simulink model "XMC_FFT2D_HDL_AIE"  (R2024a)
settings: Solver=FixedStepDiscrete  StartTime=0.0  StopTime=256*256*2  RelTol=1e-3
PreLoadFcn:
  | MRIDemo_PreloadFcn;
  | 
  | % configure hardware specifics information
  | clock_frequency = 150e6;
  | 
  | % corner bender info
  | clk = clock_frequency; %Hz
  | Tclk = 1/clk;
  | L2M = 8; % L2M=log2(M)
  | L2N = 8; % L2N=log2(N)
  | M = 2^L2M;
  | N = 2^L2N;
  | SSR = 1;
InitFcn:
  | xlEvaluateHDLBlocks('XMC_FFT2D_HDL_AIE')
undefined symbols (not defined in the file): c, gray, None, S, vsva2197, xcvc1902
libraries: hdlBasic x137, aieUtilities x3, aieDSP x2, dspxfrm3 x2, dspsrcs4 x2, simulink x1, vmcUtilities x1
(part 1 of 2)
settings Model: PauseTimes=256*254  SnapshotBufferSize=1000  SnapshotInterval=1  Creator=mmi  LastModifiedBy=sdegala
settings SolverCC: AlgebraicLoopSolver=TrustRegion
settings DataIOCC: ReturnWorkspaceOutputs=off
settings DebuggingCC: UnconnectedInputMsg=warning  UnconnectedOutputMsg=warning  UnconnectedLineMsg=warning  ArithmeticOperatorsInVariantConditions=warning
settings ModelReferenceCC: EnableRefExpFcnMdlSchedulingChecks=on
settings SFSimCC: SimUseLocalCustomCode=off  CustomCodeUndefinedFunction=UseInterfaceOnly
settings RTWCC: RTWUseLocalCustomCode=off  GPUComputeCapability=3.5  DLArmComputeVersion=19.05

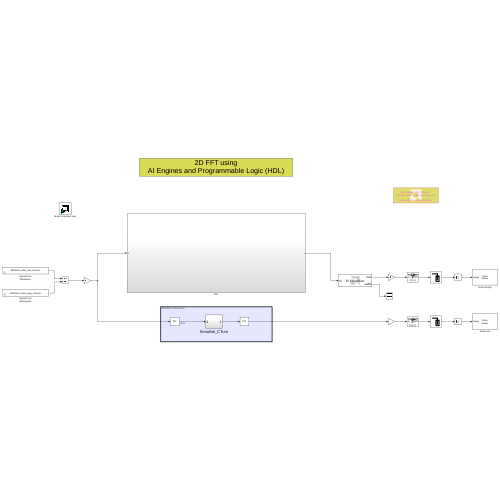
[thumbnail: Simulink's stored preview of the top-level diagram]
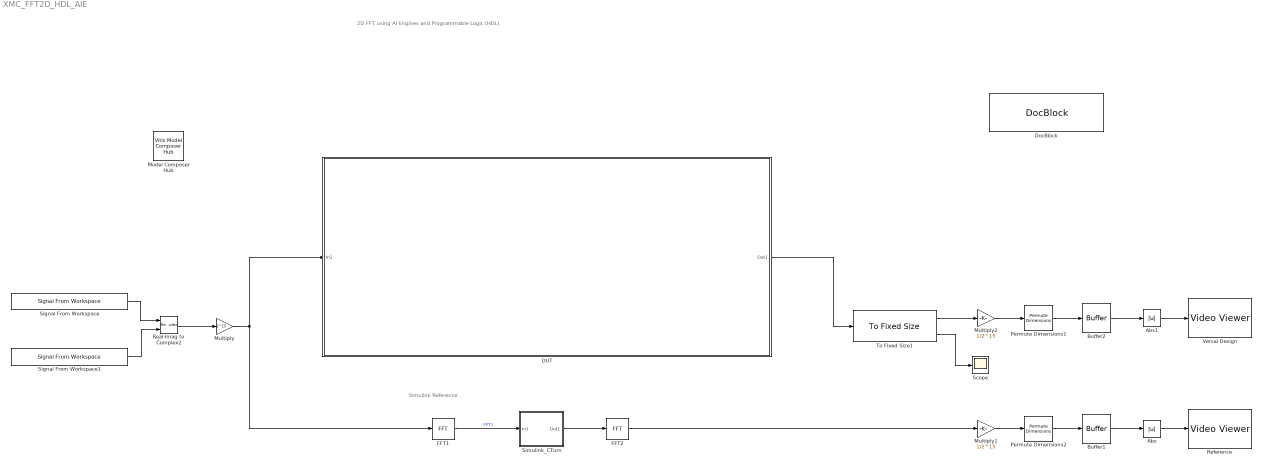
== system XMC_FFT2D_HDL_AIE ==
  note: Simulink Reference
  note: 2D FFT using
      | AI Engines and Programmable Logic (HDL)
  Abs : Abs  SaturateOnIntegerOverflow=off
  Abs1 : Abs  SaturateOnIntegerOverflow=off
  Buffer1 : Buffer  N=256  OutputFrames=off
  Buffer2 : Buffer  N=256  OutputFrames=off
  DUT : Subsystem
  DocBlock : simulink/Model-Wide Utilities/DocBlock  DocumentType=Text  mask(DocBlock){}
      content=|
      | ///////////////////////////////////////////////////////////////////////////
      | // Copyright 2021 Xilinx
      | //
      | // Licensed under the Apache License, Version 2.0 (the "License");
      | // you may not use this file except in compliance with the License.
      | // You may obtain a copy of the License at
      | //
      | // http://www.apache.org/licenses/LICENSE-2.0
      | //
      | // Unless required by applicable law or agreed to in writing, software
      | // distributed under the License is distributed on an "AS IS" BASIS,
      | // WITHOUT WARRANTIES OR CONDITIONS OF ANY KIND, either express or implied.
      | // See the License for the specific language governing permissions and
      | // limitations under the License.
      | ///////////////////////////////////////////////////////////////////////////
      mask Display:
      | xmcDrawBlockIcon();
      | disp(['{\fontsize{10pt}(c) Copyright 2021' ' Xilinx, Inc.}\newline \newline '],'texmode','on');
      | disp('{\fontsize{10pt}Licensed under the Apache License 2.0}','texmode','on');
      | disp('\newline \newline \newline{\fontsize{10pt}Double Click for Copyright Notice}','texmode','on');
  FFT1 : dspxfrm3/FFT  FFTImplementation=Auto  CompMethod=Table lookup  TableOpt=NEW  TableOptActive=Speed  BitRevOrder=off  Normalize=off  InheritFFTLength=on  FFTLength=64  WrapInput=on  roundingMode=Floor  overflowMode=off  firstCoeffDataTypeStr=Inherit: Same word length as input  firstCoeffLastDataTypeStr=Inherit: Same word length as input  prodOutputMode=Binary point scaling  prodOutputWordLength=32  prodOutputFracLength=0  prodOutputDataTypeStr=fixdt(1,32,0)  prodOutputLastDataTypeStr=fixdt(1,32,0)  accumMode=Binary point scaling  accumWordLength=48  accumFracLength=0  accumDataTypeStr=fixdt(1,48,0)  accumLastDataTypeStr=fixdt(1,48,0)  outputMode=Binary point scaling  outputWordLength=16  outputFracLength=0  outputDataTypeStr=fixdt(1,16,0)  outputMin=[]  outputMax=[]  outputLastDataTypeStr=fixdt(1,16,0)
  FFT2 : dspxfrm3/FFT  FFTImplementation=Auto  CompMethod=Table lookup  TableOpt=NEW  TableOptActive=Speed  BitRevOrder=off  Normalize=off  InheritFFTLength=on  FFTLength=64  WrapInput=on  roundingMode=Floor  overflowMode=off  firstCoeffDataTypeStr=Inherit: Same word length as input  firstCoeffLastDataTypeStr=Inherit: Same word length as input  prodOutputMode=Binary point scaling  prodOutputWordLength=32  prodOutputFracLength=0  prodOutputDataTypeStr=fixdt(1,32,0)  prodOutputLastDataTypeStr=fixdt(1,32,0)  accumMode=Binary point scaling  accumWordLength=48  accumFracLength=0  accumDataTypeStr=fixdt(1,48,0)  accumLastDataTypeStr=fixdt(1,48,0)  outputMode=Binary point scaling  outputWordLength=16  outputFracLength=0  outputDataTypeStr=fixdt(1,16,0)  outputMin=[]  outputMax=[]  outputLastDataTypeStr=fixdt(1,16,0)
  Model Composer Hub : vmcUtilities/Vitis Model Composer Hub  Tag=genX  CodeGeneration=off  SubsystemName=hdl_corner_turn  BlockHierPath=XMC_FFT2D_HDL_AIE/DUT  CompilationType=VitisCompilation  SubsystemType=DUTNode  ExportTypeV2=GenXO  AIEArrayConfig=Use entire AIE array  StartColumn=1  NumberOfColumns=1  TargetDirectory=./code  exportDesign=on  analyzeDesign=off  validateDesignOnHw=off  ExportType=Vitis Subsystem  IpVendor=xilinx.com  IpLibrary=hls  IpVersion=1.0  IpHWLanguage=Verilog  AieCompilerOptions={}  AieSimulatorOptions={}  CreateTestbench=off  TestbenchStackSize=10  RunRtlSim=off  RunCSim=off  RunAieSim=on  AieSimTimeout=50000  RunAieSimProfiling=off  LaunchVitisAnalyzer=off  PlotOutput=off  RunX86Sim=off  X86SimTimeout=10  GenHwImage=off  GenLibadfXo=on  GenHwValidationCode=on  PlatformType=Not Specified  HwSystemType=Baremetal  HwValidationTarget=hw  ProjDevice=xcvc1902-vsva2197-1LP-e-S  ProjDevicePart=xcvc1902-vsva2197-1LP-e-S  AIEType=AIE  SamplePeriod=-1  ClockFrequency=200  DataPathParallelism=1  xilinxfamily=versalaicore  part=xcvc1902  speed=-1LP-e-S  package=vsva2197  directory=./code/ip/hdl_corner_turn/src  testbench=on  incr_netlist=off  synthesis_tool=Vivado  clock_wrapper=Clock Enables  dbl_ovrd=According to Block Masks  dcm_input_clock_period=10  sysclk_period=10  simulink_period=1  eval_field=0  IPInfoJsonString="{\"DUTSubsystemName\":\"DUT\",\"HDLSubsystem\":{\"SubsystemName\":\"hdl_corner_turn\",\"IPName\":\"XMC_FFT2D_HDL_AIE\",\"IPLibrary\":\"SysGen\",\"IPVendor\":\"User Company\",\"IPVersion\":\"1.0\",\"TargetDirectory\":\"./code\",\"SubsystemDir\":\"./code/ip/hdl_corner_turn\",\"FreqHz\":\"100000000\"},\"SubsystemTag\":\"DUTNode\",\"AIESubsystem\":{\"SubsystemName\":\"aie_fft\",\"TargetDirectory\":\"./code\",\"AIEArrayConfig\":\"Use entire AIE array\",\"StartColumn\":\"1\",\"NumberOfColumns\":\"1\"}}"  LogFileName=/proj/xhdhdstaff5/sdegala/Head1/HEAD/ModelComposer_Sept16/Vitis_Model_Composer/Examples/AIENGINE_plus_PL/AIE_HDL/FFT2D/code/model_composer.log  NThreads=4  IPConfigFile=/tmp/vmctmp-7771901812203365421/XMC_FFT2D_HDL_AIE_ipconfig.json
  Multiply : Gain  Gain=2^15  OutDataTypeStr=int16
  Multiply1 : Gain  Gain=1/2^15  OutDataTypeStr=single
  Multiply2 : Gain  Gain=1/2^15  OutDataTypeStr=single
  Permute Dimensions1 : PermuteDimensions
  Permute Dimensions2 : PermuteDimensions
  Real-Imag to Complex2 : RealImagToComplex
  Reference : VideoViewer  Description=Simulink MRI Display  colormapValue=gray(256)  FigPos=[1133 905 574 478]
  Scope : Scope
  Signal From Workspace : dspsrcs4/Signal From Workspace  X=MRIDemo_data_real_channel  Ts=1  nsamps=256  OutputAfterFinalValue=Setting to zero  ignoreOrWarnInputAndFrameLengths=off  OutputFrames=off
  Signal From Workspace1 : dspsrcs4/Signal From Workspace  X=MRIDemo_data_imag_channel  Ts=1  nsamps=256  OutputAfterFinalValue=Setting to zero  ignoreOrWarnInputAndFrameLengths=off  OutputFrames=off
  Simulink_CTurn : Subsystem
  To Fixed Size1 : aieUtilities/To Fixed Size  Mode=Produce a valid output signal  OutputSize=256  CopyMethod=Buffer samples to form output  HasStatusOutput=off
  Versal Design : VideoViewer  Description=Simulink MRI Display  colormapValue=gray(256)  FigPos=[1062 805 703 270]
  wires:
  Real-Imag to Complex2/1 -> Multiply/1
  Signal From Workspace/1 -> Real-Imag to Complex2/1
  Signal From Workspace1/1 -> Real-Imag to Complex2/2
  Multiply1/1 -> Permute Dimensions2/1
  Abs/1 -> Reference/1
  Permute Dimensions2/1 -> Buffer1/1
  Buffer1/1 -> Abs/1
  Multiply/1 -> DUT/1(In1), FFT1/1
  FFT1/1 -> Simulink_CTurn/1(In1)  "FFT1"
  FFT2/1 -> Multiply1/1
  Simulink_CTurn/1(Out1) -> FFT2/1
  Abs1/1 -> Versal Design/1
  Buffer2/1 -> Abs1/1
  Permute Dimensions1/1 -> Buffer2/1
  Multiply2/1 -> Permute Dimensions1/1
  To Fixed Size1/1 -> Multiply2/1
  To Fixed Size1/2 -> Scope/1
  DUT/1(Out1) -> To Fixed Size1/1

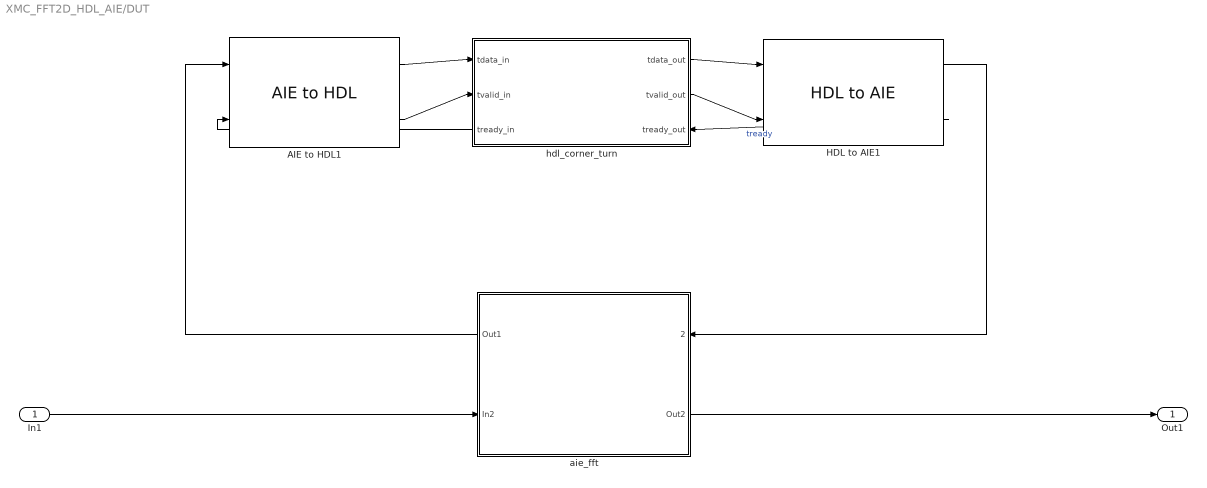
== system XMC_FFT2D_HDL_AIE/DUT ==
  In1 : Inport
  AIE to HDL1 : aieUtilities/AIE to HDL  OutDataType=uint32  OutSampleTime=1
      link override AIE to HDL_tready: inherit_from_input=on  hdl_port=on  rows=1  columns=1  UseAsDAC=off  DACChannel='1'  interface=None  automatic_assignment=on  address_offset=hex2dec('00')  intf_name=''  intf_description=''  timing_constraint=None  locs_specified=off  LOCs={}  io_standard={}
      link override AIE to HDL_tready: infoedit="Gateway out block.  Converts Xilinx fixed-point or floating-point type inputs into ouputs of type Simulink integer, single, double, or fixed-point.<br><br>Hardware notes:  In hardware these blocks become top level output ports or are discarded, depending on how they are configured."
  HDL to AIE1 : aieUtilities/HDL to AIE  InDataType=uint32  OutDataType=int16 (c)  OutSampleTime=1  SamplesPerFrame=256  RateReduceFactor=1  ManuallySpecifyOutSampleTime=on
  aie_fft : Subsystem
      settings: PortSchema="{\"entries\":[{\"content\":{\"sides\":[{\"content\":{\"connectorIds\":[\"Out2\",\"In1\"]},\"type\":\"ConnectorPlacement.EquallySpacedRectSide\",\"uuid\":\"ba116f73-e116-40b3-b2e5-304cba4df7e1\"},{\"content\":{\"connectorIds\":[\"In2\",\"Out1\"],\"side\":\"RIGHT\"},\"type\":\"ConnectorPlacement.EquallySpacedRectSide\",\"uuid\":\"f8ace37c-ffb0-4f56-a1b3-7eeef7565cfd\"},{\"content\":{\"connectorIds\":[],\"side\":\"TOP\"},\"type\":\"ConnectorPlacement.EquallySpacedRectSide\",\"uuid\":\"698d2e0a-1e8b-402b-bc99-cd34e1f9cd41\"}]},\"type\":\"ConnectorPlacement.EquallySpacedConnector\",\"uuid\":\"c9271cff-0d68-4ac4-bc57-5327e013a37e\"}],\"packageUris\":[\"http://schema.mathworks.com/mf0/Connector/R2020b\"],\"version\":\"1.0\"}"
  hdl_corner_turn : Subsystem
      settings: PortSchema="{\"entries\":[{\"content\":{\"sides\":[{\"content\":{\"connectorIds\":[\"In1\",\"In2\",\"Out3\"]},\"type\":\"ConnectorPlacement.EquallySpacedRectSide\",\"uuid\":\"096cfc4a-45cf-495e-9dad-5ec39c034de1\"},{\"content\":{\"connectorIds\":[\"Out1\",\"Out2\",\"In3\"],\"side\":\"RIGHT\"},\"type\":\"ConnectorPlacement.EquallySpacedRectSide\",\"uuid\":\"c2f58c53-17c1-4e0f-8fe6-4ca31b4ae7e7\"},{\"content\":{\"connectorIds\":[],\"side\":\"TOP\"},\"type\":\"ConnectorPlacement.EquallySpacedRectSide\",\"uuid\":\"fc0a0e48-62d9-4bc4-85b8-28883543f418\"}]},\"type\":\"ConnectorPlacement.EquallySpacedConnector\",\"uuid\":\"4d40c623-5fa9-4077-a912-8400e8a8f04d\"}],\"packageUris\":[\"http://schema.mathworks.com/mf0/Connector/R2020b\"],\"version\":\"1.0\"}"
  Out1 : Outport
  wires:
  hdl_corner_turn/3(tready_in) -> AIE to HDL1/2
  AIE to HDL1/2 -> hdl_corner_turn/2(tvalid_in)
  hdl_corner_turn/2(tvalid_out) -> HDL to AIE1/2
  aie_fft/1(Out2) -> Out1/1
  HDL to AIE1/2 -> hdl_corner_turn/3(tready_out)  "tready"
  In1/1 -> aie_fft/1(In2)
  AIE to HDL1/1 -> hdl_corner_turn/1(tdata_in)
  hdl_corner_turn/1(tdata_out) -> HDL to AIE1/1
  HDL to AIE1/1 -> aie_fft/2(" ")
  aie_fft/2(Out1) -> AIE to HDL1/1

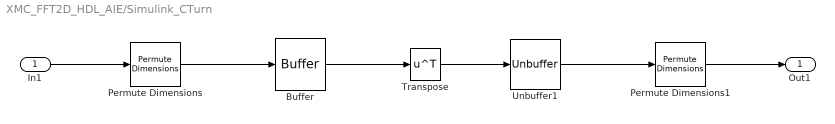
== system XMC_FFT2D_HDL_AIE/Simulink_CTurn ==
  In1 : Inport
  Buffer : Buffer  N=256  OutputFrames=off
  Permute Dimensions : PermuteDimensions
  Permute Dimensions1 : PermuteDimensions
  Transpose : Math  Operator=transpose  SignedPower=on
  Unbuffer1 : Unbuffer
  Out1 : Outport  VectorParamsAs1DForOutWhenUnconnected=off
  wires:
  Permute Dimensions/1 -> Buffer/1
  Transpose/1 -> Unbuffer1/1
  Buffer/1 -> Transpose/1
  In1/1 -> Permute Dimensions/1
  Unbuffer1/1 -> Permute Dimensions1/1
  Permute Dimensions1/1 -> Out1/1

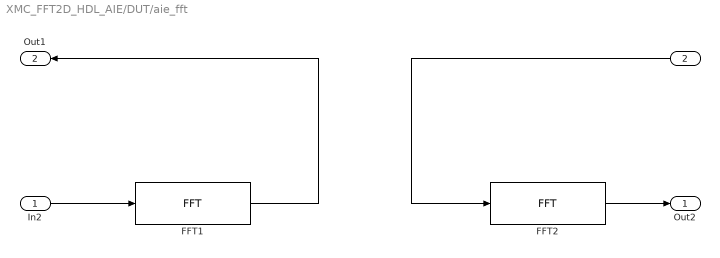
== system XMC_FFT2D_HDL_AIE/DUT/aie_fft ==
  In2 : Inport
  " " : Inport  Port=2
  FFT1 : aieDSP/FFT  AIE_VARIANT=1  data_type=cint16  data_out_type=cint16  twiddle_type=cint16  point_size=256  input_window_size=256  shift_val=0  rnd_mode=Round to positive infinity  sat_mode=0-None  ssr=1  twiddle_mode=0  use_ssr_widget_kernels=off  casc_length=1  transform_fft_nifft=1  TP_API=0  TP_DYN_PT_SIZE=0  blockJsonConstraints=[]  blockJsonConstraintsInternal="{\"type\":\"constraint\",\"constraintType\":\"coreUtilization\",\"sid\":\"82030:fft_graph.FFTwinproc.m_fftKernels[0]\",\"lhs\":{\"type\":\"runtimeRatio\",\"args\":{\"type\":\"kernel\",\"name\":\"XMC_FFT2D_HDL_AIE/Versal Desgin/aie_fft/FFT1\",\"sid\":\"82030:fft_graph.FFTwinproc.m_fftKernels[0]\"}},\"rhs\":{\"type\":\"evaluable\",\"expr\":\"0.9\",\"value\":0.9},\"equality\":true}"  spec=vmc_fft.json  SerializedMaskParamNames=[]  SerializedMaskParamValues=[]  SerializedMaskParamVisibilities=[]  block_type=FFT  SerializedMaskParamDataypes=uint|typename|typename|typename|uint|uint|uint|uint|uint|uint|uint|uint|uint|uint|uint|uint  SerializedMaskParamEnumStrArr=0|0|0|0|0|0|0|Round to positive infinity,Round to negative infinity,Round symmetrical to infinity,Round symmetrical to zero,Round convergent to even,Round convergent to odd|0-None,1-Asymmetric,3-Symmetric|0|0|0|0|0|0|0  SerializedMaskParamEnumValArr=0|0|0|0|0|0|0|2,3,4,5,6,7|0,1,3|0|0|0|0|0|0|0  SerializedMaskParamVectorArr=0|0|0|0|0|0|0|0|0|0|0|0|0|0|0|0  SerializedMaskParamKeys=AIE_VARIANT|TT_DATA|TT_OUT_DATA|TT_TWIDDLE|TP_POINT_SIZE|TP_WINDOW_VSIZE|TP_SHIFT|TP_RND|TP_SAT|TP_PARALLEL_POWER|TP_TWIDDLE_MODE|TP_USE_WIDGETS|TP_CASC_LEN|TP_FFT_NIFFT|TP_API|TP_DYN_PT_SIZE
  FFT2 : aieDSP/FFT  AIE_VARIANT=1  data_type=cint16  data_out_type=cint16  twiddle_type=cint16  point_size=256  input_window_size=256  shift_val=0  rnd_mode=Round to positive infinity  sat_mode=0-None  ssr=1  twiddle_mode=0  use_ssr_widget_kernels=off  casc_length=1  transform_fft_nifft=1  TP_API=0  TP_DYN_PT_SIZE=0  blockJsonConstraints=[]  blockJsonConstraintsInternal="{\"type\":\"constraint\",\"constraintType\":\"coreUtilization\",\"sid\":\"82031:fft_graph.FFTwinproc.m_fftKernels[0]\",\"lhs\":{\"type\":\"runtimeRatio\",\"args\":{\"type\":\"kernel\",\"name\":\"XMC_FFT2D_HDL_AIE/Versal Desgin/aie_fft/FFT2\",\"sid\":\"82031:fft_graph.FFTwinproc.m_fftKernels[0]\"}},\"rhs\":{\"type\":\"evaluable\",\"expr\":\"0.9\",\"value\":0.9},\"equality\":true}"  spec=vmc_fft.json  SerializedMaskParamNames=[]  SerializedMaskParamValues=[]  SerializedMaskParamVisibilities=[]  block_type=FFT  SerializedMaskParamDataypes=uint|typename|typename|typename|uint|uint|uint|uint|uint|uint|uint|uint|uint|uint|uint|uint  SerializedMaskParamEnumStrArr=0|0|0|0|0|0|0|Round to positive infinity,Round to negative infinity,Round symmetrical to infinity,Round symmetrical to zero,Round convergent to even,Round convergent to odd|0-None,1-Asymmetric,3-Symmetric|0|0|0|0|0|0|0  SerializedMaskParamEnumValArr=0|0|0|0|0|0|0|2,3,4,5,6,7|0,1,3|0|0|0|0|0|0|0  SerializedMaskParamVectorArr=0|0|0|0|0|0|0|0|0|0|0|0|0|0|0|0  SerializedMaskParamKeys=AIE_VARIANT|TT_DATA|TT_OUT_DATA|TT_TWIDDLE|TP_POINT_SIZE|TP_WINDOW_VSIZE|TP_SHIFT|TP_RND|TP_SAT|TP_PARALLEL_POWER|TP_TWIDDLE_MODE|TP_USE_WIDGETS|TP_CASC_LEN|TP_FFT_NIFFT|TP_API|TP_DYN_PT_SIZE
  Out2 : Outport
  Out1 : Outport  Port=2
  wires:
  FFT2/1 -> Out2/1
  " "/1 -> FFT2/1
  FFT1/1 -> Out1/1
  In2/1 -> FFT1/1

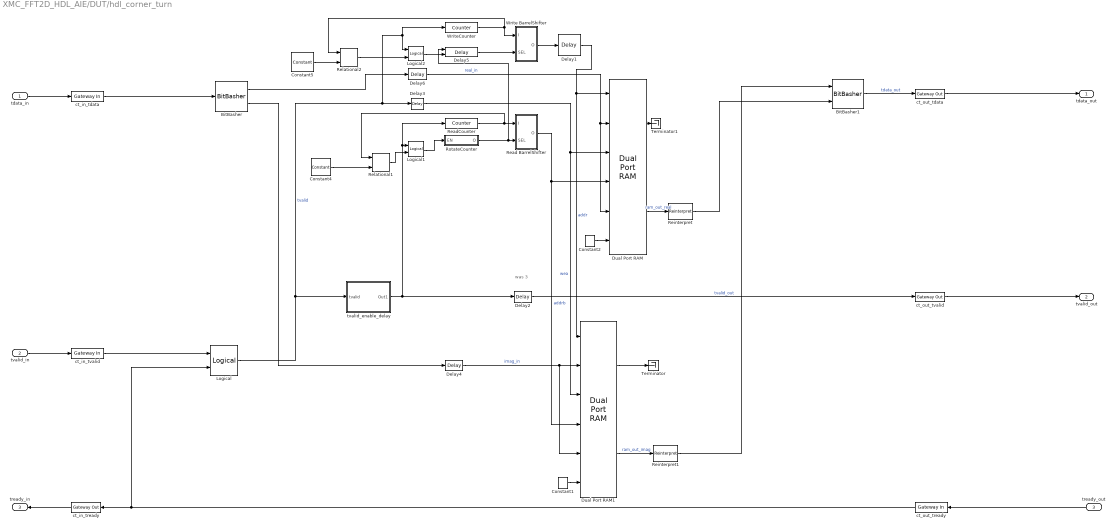
== system XMC_FFT2D_HDL_AIE/DUT/hdl_corner_turn ==
  note: was 3
  tdata_in : Inport
  tvalid_in : Inport  Port=2
  tready_out : Inport  Port=3
  BitBasher : hdlBasic/BitBasher  bitexpr=|  display_expr=off  sr_1=re  arith_type1="Signed  (2's comp)"  bin_pt1=0  sr_2=im  arith_type2="Signed  (2's comp)"  bin_pt2=0  sr_3=3  arith_type3=Unsigned  bin_pt3=0  sr_4=4  arith_type4=Unsigned  bin_pt4=0  XmcBlockStatus=1  maskContainerNames=group1  block_type=bitbasher  block_config=sysgen:BitBasher_config
      | re={cplx_in[15:0]};
      | im={cplx_in[31:16]};
  BitBasher1 : hdlBasic/BitBasher  bitexpr=cplx_out={im[15:0], re[15:0]};  display_expr=off  sr_1=cplx_out  arith_type1=Unsigned  bin_pt1=0  sr_2=im  arith_type2=Unsigned  bin_pt2=0  sr_3=3  arith_type3=Unsigned  bin_pt3=0  sr_4=4  arith_type4=Unsigned  bin_pt4=0  XmcBlockStatus=1  maskContainerNames=group1  block_type=bitbasher  block_config=sysgen:BitBasher_config
  Constant1 : hdlBasic/Constant  const=0  gui_display_data_type=Boolean  arith_type=Boolean  n_bits=40  bin_pt=20  preci_type=Single  exp_width=8  frac_width=24  explicit_period=off  period=1  XmcBlockStatus=1  maskContainerNames=tabcontainer1  block_type=constant  block_config=sysgen:Constant_config
  Constant2 : hdlBasic/Constant  const=0  gui_display_data_type=Boolean  arith_type=Boolean  n_bits=40  bin_pt=20  preci_type=Single  exp_width=8  frac_width=24  explicit_period=off  period=1  XmcBlockStatus=1  maskContainerNames=tabcontainer1  block_type=constant  block_config=sysgen:Constant_config
  Constant4 : hdlBasic/Constant  const=2^(L2M+L2N)-1  gui_display_data_type=Fixed-point  arith_type=Unsigned  n_bits=L2M+L2N  bin_pt=0  preci_type=Single  exp_width=8  frac_width=24  explicit_period=off  period=1  XmcBlockStatus=1  maskContainerNames=tabcontainer1  block_type=constant  block_config=sysgen:Constant_config
  Constant5 : hdlBasic/Constant  const=2^(L2M+L2N)-1  gui_display_data_type=Fixed-point  arith_type=Unsigned  n_bits=L2M+L2N  bin_pt=0  preci_type=Single  exp_width=8  frac_width=24  explicit_period=off  period=1  XmcBlockStatus=1  maskContainerNames=tabcontainer1  block_type=constant  block_config=sysgen:Constant_config
  Delay1 : hdlBasic/Delay  rst=off  en=off  latency=1  reg_retiming=off  XmcBlockStatus=1  maskContainerNames=group1  block_type=delay  block_config=sysgen:Delay_config
  Delay2 : hdlBasic/Delay  rst=off  en=off  latency=3  reg_retiming=off  XmcBlockStatus=1  maskContainerNames=group1  block_type=delay  block_config=sysgen:Delay_config
  Delay3 : hdlBasic/Delay  rst=off  en=off  latency=2  reg_retiming=off  XmcBlockStatus=1  maskContainerNames=group1  block_type=delay  block_config=sysgen:Delay_config
  Delay4 : hdlBasic/Delay  rst=off  en=off  latency=2  reg_retiming=off  XmcBlockStatus=1  maskContainerNames=group1  block_type=delay  block_config=sysgen:Delay_config
  Delay5 : hdlBasic/Delay  rst=off  en=on  latency=1  reg_retiming=off  XmcBlockStatus=1  maskContainerNames=group1  block_type=delay  block_config=sysgen:Delay_config
  Delay6 : hdlBasic/Delay  rst=off  en=off  latency=2  reg_retiming=off  XmcBlockStatus=1  maskContainerNames=group1  block_type=delay  block_config=sysgen:Delay_config
  Dual Port RAM : hdlBasic/Dual Port RAM  depth=2^L2M*2^L2N  initVector=zeros(2^L2M*2^L2N,1)  distributed_mem=Block RAM  init_a=0  init_b=0  rst_a=off  rst_b=off  en_a=off  en_b=off  latency=2  write_mode_A=Read After Write  write_mode_B=Read After Write  explicit_period=[]  period=[]  simulation_type=fast_sim  XmcBlockStatus=1  maskContainerNames=tabcontainer1  block_type=dpram  block_config=sysgen:Dpram_config  optimize=Area
      settings: infoedit=[]
  Dual Port RAM1 : hdlBasic/Dual Port RAM  depth=2^L2M*2^L2N  initVector=zeros(2^L2M*2^L2N,1)  distributed_mem=Block RAM  init_a=0  init_b=0  rst_a=off  rst_b=off  en_a=off  en_b=off  latency=2  write_mode_A=Read After Write  write_mode_B=Read After Write  explicit_period=[]  period=[]  simulation_type=fast_sim  XmcBlockStatus=1  maskContainerNames=tabcontainer1  block_type=dpram  block_config=sysgen:Dpram_config  optimize=Area
      settings: infoedit=[]
  Logical : hdlBasic/Logical  logical_function=AND  inputs=2  en=off  latency=0  precision=Full  arith_type=Unsigned  n_bits=16  bin_pt=0  align_bp=on  overflow=[]  quantization=[]  XmcBlockStatus=1  maskContainerNames=tabcontainer1  block_type=logical  block_config=sysgen:Logical_config
  Logical1 : hdlBasic/Logical  logical_function=AND  inputs=2  en=off  latency=0  precision=Full  arith_type=Unsigned  n_bits=16  bin_pt=0  align_bp=on  overflow=[]  quantization=[]  XmcBlockStatus=1  maskContainerNames=tabcontainer1  block_type=logical  block_config=sysgen:Logical_config
  Logical2 : hdlBasic/Logical  logical_function=AND  inputs=2  en=off  latency=0  precision=Full  arith_type=Unsigned  n_bits=16  bin_pt=0  align_bp=on  overflow=[]  quantization=[]  XmcBlockStatus=1  maskContainerNames=tabcontainer1  block_type=logical  block_config=sysgen:Logical_config
  Read BarrelShifter : Subsystem  mask{barrel_length=L2M+L2N}
      mask prompts: barrel_length "Barrel Length"
      mask init:
      | %%%%%%%%%%%%%%%%%%%%%%%%%%%%%%%%%%%%%%%%%%%%%%%%%%%%%
      | % Parametric Barrel Shifter Mask Initialization Script
      | % 18DEC2017: Creation
      | %%%%%%%%%%%%%%%%%%%%%%%%%%%%%%%%%%%%%%%%%%%%%%%%%%%%%
      | this=gcb;
      | 
      | %%%%%%%%%%%%%%%%%%%%%%%%%%%%%%%%%%%%%%%%%%%%%%%%%%%%%
      | % Delete wires and certain blocks; retain IO ports so parent
      | % mask block will not require re-connection
      | %%%%%%%%%%%%%%%%%%%%%%%%%%%%%%%%%%%%%%%%%%%%%%%%%%%%%
      | 
      | % delete all blocks except for d1 and q1
      | allblocks = find_system(this, 'LookUnderMasks','on','SearchDepth',1);
      | 
      | ToKeep = {'I';'O';'SEL';'Mux';'RotateLeft1'};
      | 
      | %// add systemname to strings
      | ToKeep = strcat(repmat({[this  '/']},numel(ToKeep),1), ToKeep);
      | 
      | %// create mask
      | ToDelete = setdiff(allblocks,ToKeep);
      | %// filter out main system
      | ToDelete = setxor(ToDelete,this);
      | 
      | cellfun(@(x) delete_block(x),ToDelete)
      | 
      | % delete lines
      | L = find_system(this,'LookUnderMasks','on','SearchDepth',1,'FindAll','on','type','line');
      | delete_line(L(1:end));
      | 
      | %%%%%%%%%%%%%%%%%%%%%%%%%%%%%%%%%%%%%%%%%%%%%%%%%%%%%%
      | % instantiate RotateLeft blocks and configure
      | %%%%%%%%%%%%%%%%%%%%%%%%%%%%%%%%%%%%%%%%%%%%%%%%%%%%%%
      | blockName1 = strcat(this,'/RotateLeft1');
      | x_loc = 70;
      | y_loc = 70;
      | for i = 2:barrel_length-1
      |     blockName = strcat(this,'/RotateLeft',num2str(i));
      |     blockHandle = add_block(blockName1,blockName, 'position',[x_loc,y_loc,x_loc+60,y_loc+20], ...
      |         'NB',num2str(i));
      |     y_loc = y_loc + 40;
      | end
      | 
      | %%%%%%%%%%%%%%%%%%%%%%%%%%%%%%%%%%%%%%%%%%%%%%%%%%%%%%
      | % Set mux parameters
      | %%%%%%%%%%%%%%%%%%%%%%%%%%%%%%%%%%%%%%%%%%%%%%%%%%%%%%
      | 
      | myMux = strcat(this,'/Mux');
      | set_param(myMux, 'inputs', barrel_length-2);
      | 
      | %%%%%%%%%%%%%%%%%%%%%%%%%%%%%%%%%%%%%%%%%%%%%%%%%%%%%%
      | % wires
      | %%%%%%%%%%%%%%%%%%%%%%%%%%%%%%%%%%%%%%%%%%%%%%%%%%%%%%
      | 
      | % RotateLeft to mux
      | 
      | h_myMux = get_param(myMux,'PortHandles');
      | 
      | for i = 1:barrel_length-1  
      |   blockName = strcat(this,'/RotateLeft',num2str(i));
      |   h_RotateLeft =  get_param(blockName,'PortHandles');
      |   add_line(this,{h_RotateLeft.Outport} ,{h_myMux.Inport(i+2)},'autorouting','on');
      | end
      | 
      | % mux to outport
      | h_myOutport = get_param(strcat(this,'/O'), 'PortHandles');
      | 
      | add_line(this,{h_myMux.Outport} ,{h_myOutport.Inport},'autorouting','on');
      | 
      | % inport to RotateLeft
      | h_myInport = get_param(strcat(this,'/I'), 'PortHandles');
      | 
      | for i = 1:barrel_length-1  
      |   blockName = strcat(this,'/RotateLeft',num2str(i));
      |   h_RotateLeft =  get_param(blockName,'PortHandles');
      |   add_line(this,{h_myInport.Outport} ,{h_RotateLeft.Inport},'autorouting','on');
      | end
      | 
      | % inport to mux
      | add_line(this,{h_myInport.Outport} ,{h_myMux.Inport(2)},'autorouting','on');
      | 
      | % SEL to mux
      | h_mySEL = get_param(strcat(this,'/SEL'), 'PortHandles');
      | add_line(this,{h_mySEL.Outport} ,{h_myMux.Inport(1)},'autorouting','on');
  ReadCounter : hdlBasic/Counter  cnt_type=Free running  cnt_to=Inf  operation=Up  start_count=0  cnt_by_val=1  arith_type=Unsigned  n_bits=L2M+L2N  bin_pt=0  load_pin=off  rst=off  en=on  explicit_period=Explicit  period=1  use_behavioral_HDL=off  implementation=Fabric  XmcBlockStatus=1  maskContainerNames=group1  block_type=counter  block_config=sysgen:Counter_config  block_width=531  block_height=1023
  Reinterpret : hdlBasic/Reinterpret  force_arith_type=on  arith_type=Unsigned  force_bin_pt=off  bin_pt=0  XmcBlockStatus=1  maskContainerNames=group1  block_type=reinterpret  block_config=sysgen:Reinterpret_config
  Reinterpret1 : hdlBasic/Reinterpret  force_arith_type=on  arith_type=Unsigned  force_bin_pt=off  bin_pt=0  XmcBlockStatus=1  maskContainerNames=group1  block_type=reinterpret  block_config=sysgen:Reinterpret_config
  Relational1 : hdlBasic/Relational  mode=a=b  op_type=Bool  en=off  latency=0  XmcBlockStatus=1  maskContainerNames=tabcontainer1  block_type=relational  block_config=sysgen:Relational_config
  Relational2 : hdlBasic/Relational  mode=a=b  op_type=Bool  en=off  latency=0  XmcBlockStatus=1  maskContainerNames=tabcontainer1  block_type=relational  block_config=sysgen:Relational_config
  RotateCounter : Subsystem  mask{L2M=L2M, L2N=L2N}
  Terminator : Terminator
  Terminator1 : Terminator
  Write BarrelShifter : Subsystem  mask{barrel_length=L2M+L2N}
      mask prompts: barrel_length "Barrel Length"
      mask init: same as XMC_FFT2D_HDL_AIE/DUT/hdl_corner_turn/Read BarrelShifter
  WriteCounter : hdlBasic/Counter  cnt_type=Free running  cnt_to=Inf  operation=Up  start_count=0  cnt_by_val=1  arith_type=Unsigned  n_bits=L2M+L2N  bin_pt=0  load_pin=off  rst=off  en=on  explicit_period=Explicit  period=1  use_behavioral_HDL=off  implementation=Fabric  XmcBlockStatus=1  maskContainerNames=group1  block_type=counter  block_config=sysgen:Counter_config  block_width=531  block_height=1023
  ct_in_tdata : hdlBasic/Gateway In  gui_display_data_type=Fixed-point  arith_type=Unsigned  n_bits=32  bin_pt=0  preci_type=Single  exp_width=8  frac_width=24  rows=1  columns=1  quantization="Round  (unbiased: +/- Inf)"  overflow=Saturate  period=1  UseAsADC=off  ADCChannel='1'  interface=None  automatic_assignment=on  address_offset=hex2dec('00')  intf_name=''  intf_description=''  default_value=0  timing_constraint=None  locs_specified=off  LOCs={}  io_standard={}  inherit_from_input=off  hdl_port=on  XmcBlockStatus=1  maskContainerNames=group4  block_type=gatewayin  block_config=sysgen:gateway_in_config  block_width_w=590  block_height_w=620  block_width=640  block_height=850
  ct_in_tready : hdlBasic/Gateway Out  inherit_from_input=on  bool_to_boolean=off  hdl_port=on  rows=1  columns=1  UseAsDAC=off  DACChannel='1'  interface=None  automatic_assignment=on  address_offset=hex2dec('00')  intf_name=''  intf_description=''  timing_constraint=None  locs_specified=off  LOCs={}  io_standard={}  XmcBlockStatus=1  maskContainerNames=group4  block_type=gatewayout  block_config=sysgen:gateway_out_config  block_width_w=590  block_height_w=620  block_width=620  block_height=750
  ct_in_tvalid : hdlBasic/Gateway In  gui_display_data_type=Boolean  arith_type=Boolean  n_bits=16  bin_pt=14  preci_type=Single  exp_width=8  frac_width=24  rows=1  columns=1  quantization="Round  (unbiased: +/- Inf)"  overflow=Saturate  period=1  UseAsADC=off  ADCChannel='1'  interface=None  automatic_assignment=on  address_offset=hex2dec('00')  intf_name=''  intf_description=''  default_value=0  timing_constraint=None  locs_specified=off  LOCs={}  io_standard={}  inherit_from_input=off  hdl_port=on  XmcBlockStatus=1  maskContainerNames=group4  block_type=gatewayin  block_config=sysgen:gateway_in_config  block_width_w=590  block_height_w=620  block_width=640  block_height=850
  ct_out_tdata : hdlBasic/Gateway Out  inherit_from_input=on  bool_to_boolean=off  hdl_port=on  rows=1  columns=1  UseAsDAC=off  DACChannel='1'  interface=None  automatic_assignment=on  address_offset=hex2dec('00')  intf_name=''  intf_description=''  timing_constraint=None  locs_specified=off  LOCs={}  io_standard={}  XmcBlockStatus=1  maskContainerNames=group4  block_type=gatewayout  block_config=sysgen:gateway_out_config  block_width_w=590  block_height_w=620  block_width=620  block_height=750
  ct_out_tready : hdlBasic/Gateway In  gui_display_data_type=Boolean  arith_type=Boolean  n_bits=16  bin_pt=14  preci_type=Single  exp_width=8  frac_width=24  rows=1  columns=1  quantization="Round  (unbiased: +/- Inf)"  overflow=Saturate  period=1  UseAsADC=off  ADCChannel='1'  interface=None  automatic_assignment=on  address_offset=hex2dec('00')  intf_name=''  intf_description=''  default_value=0  timing_constraint=None  locs_specified=off  LOCs={}  io_standard={}  inherit_from_input=off  hdl_port=on  XmcBlockStatus=1  maskContainerNames=group4  block_type=gatewayin  block_config=sysgen:gateway_in_config  block_width_w=590  block_height_w=620  block_width=640  block_height=850
  ct_out_tvalid : hdlBasic/Gateway Out  inherit_from_input=on  bool_to_boolean=off  hdl_port=on  rows=1  columns=1  UseAsDAC=off  DACChannel='1'  interface=None  automatic_assignment=on  address_offset=hex2dec('00')  intf_name=''  intf_description=''  timing_constraint=None  locs_specified=off  LOCs={}  io_standard={}  XmcBlockStatus=1  maskContainerNames=group4  block_type=gatewayout  block_config=sysgen:gateway_out_config  block_width_w=590  block_height_w=620  block_width=620  block_height=750
  tvalid_enable_delay : Subsystem
  tdata_out : Outport
  tvalid_out : Outport  Port=2
  tready_in : Outport  Port=3
  wires:
  Constant4/1 -> Relational1/2
  RotateCounter/1(O) -> Delay5/1, Read BarrelShifter/2(SEL)
  Constant1/1 -> Dual Port RAM1/6
  Reinterpret/1 -> BitBasher1/2
  Delay5/1 -> Write BarrelShifter/2(SEL)
  Relational1/1 -> Logical1/2
  Logical2/1 -> Delay5/2
  Constant5/1 -> Relational2/2
  ReadCounter/1 -> Read BarrelShifter/1(I), Relational1/1
  Dual Port RAM/2 -> Reinterpret/1  "ram_out_real"
  Read BarrelShifter/1(O) -> Dual Port RAM/4, Dual Port RAM1/4  "addrb"
  WriteCounter/1 -> Write BarrelShifter/1(I), Relational2/1
  Logical1/1 -> RotateCounter/1(EN)
  Delay4/1 -> Dual Port RAM1/5, Dual Port RAM1/2  "imag_in"
  BitBasher/2 -> Delay4/1
  Delay6/1 -> Dual Port RAM/5, Dual Port RAM/2  "real_in"
  tdata_in/1 -> ct_in_tdata/1
  Delay3/1 -> Dual Port RAM1/3, Dual Port RAM/3  "wea"
  Delay2/1 -> ct_out_tvalid/1  "tvalid_out"
  Dual Port RAM/1 -> Terminator1/1
  BitBasher1/1 -> ct_out_tdata/1  "tdata_out"
  Logical/1 -> Logical2/1, WriteCounter/1, Delay3/1, tvalid_enable_delay/1(tvalid)  "tvalid"
  Constant2/1 -> Dual Port RAM/6
  Dual Port RAM1/1 -> Terminator/1
  Write BarrelShifter/1(O) -> Delay1/1
  tvalid_in/1 -> ct_in_tvalid/1
  Relational2/1 -> Logical2/2
  Reinterpret1/1 -> BitBasher1/1
  tvalid_enable_delay/1(Out1) -> Delay2/1, ReadCounter/1, Logical1/1
  BitBasher/1 -> Delay6/1
  Delay1/1 -> Dual Port RAM/1, Dual Port RAM1/1  "addr"
  Dual Port RAM1/2 -> Reinterpret1/1  "ram_out_imag"
  tready_out/1 -> ct_out_tready/1
  ct_in_tdata/1 -> BitBasher/1
  ct_in_tvalid/1 -> Logical/1
  ct_out_tready/1 -> Logical/2, ct_in_tready/1
  ct_in_tready/1 -> tready_in/1
  ct_out_tvalid/1 -> tvalid_out/1
  ct_out_tdata/1 -> tdata_out/1

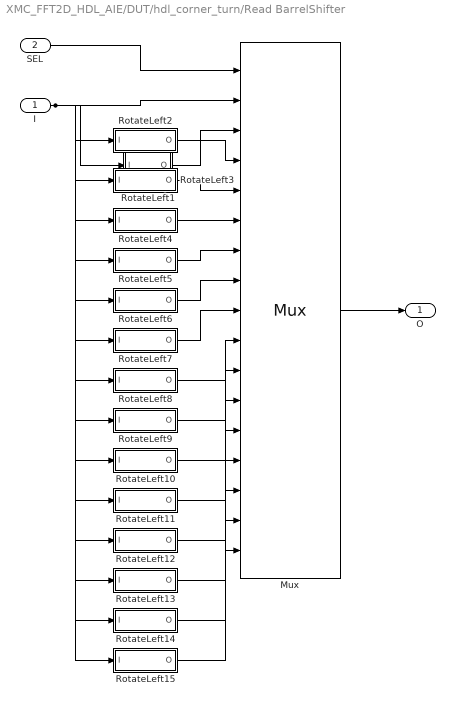
== system XMC_FFT2D_HDL_AIE/DUT/hdl_corner_turn/Read BarrelShifter ==
  I : Inport
  SEL : Inport  Port=2
  Mux : hdlBasic/Mux  inputs=16  en=off  latency=1  precision=Full  arith_type=Unsigned  n_bits=16  bin_pt=14  quantization=Truncate  overflow=Wrap  XmcBlockStatus=1  maskContainerNames=tabcontainer1  block_type=mux  block_config=sysgen:Mux_config
  RotateLeft1 : Subsystem  mask{NB=1, W=barrel_length}
      mask prompts: NB "Number of bits (cannot be 0):"; W "Width"
  RotateLeft10 : Subsystem  mask{NB=10, W=barrel_length}
      mask prompts: NB "Number of bits (cannot be 0):"; W "Width"
  RotateLeft11 : Subsystem  mask{NB=11, W=barrel_length}
      mask prompts: NB "Number of bits (cannot be 0):"; W "Width"
  RotateLeft12 : Subsystem  mask{NB=12, W=barrel_length}
      mask prompts: NB "Number of bits (cannot be 0):"; W "Width"
  RotateLeft13 : Subsystem  mask{NB=13, W=barrel_length}
      mask prompts: NB "Number of bits (cannot be 0):"; W "Width"
  RotateLeft14 : Subsystem  mask{NB=14, W=barrel_length}
      mask prompts: NB "Number of bits (cannot be 0):"; W "Width"
  RotateLeft15 : Subsystem  mask{NB=15, W=barrel_length}
      mask prompts: NB "Number of bits (cannot be 0):"; W "Width"
  RotateLeft2 : Subsystem  mask{NB=2, W=barrel_length}
      mask prompts: NB "Number of bits (cannot be 0):"; W "Width"
  RotateLeft3 : Subsystem  mask{NB=3, W=barrel_length}
      mask prompts: NB "Number of bits (cannot be 0):"; W "Width"
  RotateLeft4 : Subsystem  mask{NB=4, W=barrel_length}
      mask prompts: NB "Number of bits (cannot be 0):"; W "Width"
  RotateLeft5 : Subsystem  mask{NB=5, W=barrel_length}
      mask prompts: NB "Number of bits (cannot be 0):"; W "Width"
  RotateLeft6 : Subsystem  mask{NB=6, W=barrel_length}
      mask prompts: NB "Number of bits (cannot be 0):"; W "Width"
  RotateLeft7 : Subsystem  mask{NB=7, W=barrel_length}
      mask prompts: NB "Number of bits (cannot be 0):"; W "Width"
  RotateLeft8 : Subsystem  mask{NB=8, W=barrel_length}
      mask prompts: NB "Number of bits (cannot be 0):"; W "Width"
  RotateLeft9 : Subsystem  mask{NB=9, W=barrel_length}
      mask prompts: NB "Number of bits (cannot be 0):"; W "Width"
  O : Outport
  wires:
  RotateLeft1/1(O) -> Mux/3
  RotateLeft2/1(O) -> Mux/4
  RotateLeft3/1(O) -> Mux/5
  RotateLeft4/1(O) -> Mux/6
  RotateLeft5/1(O) -> Mux/7
  RotateLeft6/1(O) -> Mux/8
  RotateLeft7/1(O) -> Mux/9
  RotateLeft8/1(O) -> Mux/10
  RotateLeft9/1(O) -> Mux/11
  RotateLeft10/1(O) -> Mux/12
  RotateLeft11/1(O) -> Mux/13
  RotateLeft12/1(O) -> Mux/14
  RotateLeft13/1(O) -> Mux/15
  RotateLeft14/1(O) -> Mux/16
  RotateLeft15/1(O) -> Mux/17
  Mux/1 -> O/1
  I/1 -> RotateLeft1/1(I), RotateLeft2/1(I), RotateLeft3/1(I), RotateLeft4/1(I), RotateLeft5/1(I), RotateLeft6/1(I), RotateLeft7/1(I), RotateLeft8/1(I), RotateLeft9/1(I), RotateLeft10/1(I), RotateLeft11/1(I), RotateLeft12/1(I), RotateLeft13/1(I), RotateLeft14/1(I), RotateLeft15/1(I), Mux/2
  SEL/1 -> Mux/1

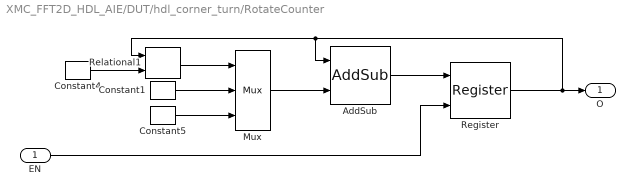
== system XMC_FFT2D_HDL_AIE/DUT/hdl_corner_turn/RotateCounter ==
  EN : Inport
  AddSub : hdlBasic/AddSub  mode=Addition  use_carryin=off  use_carryout=off  en=off  latency=0  precision=User Defined  arith_type=Unsigned  n_bits=ceil(log2(L2M+L2N))  bin_pt=0  quantization=Truncate  overflow=Wrap  use_behavioral_HDL=off  hw_selection=Fabric  pipelined=off  XmcBlockStatus=1  maskContainerNames=tabcontainer1  block_type=addsub  block_config=sysgen:Addsub_config
  Constant1 : hdlBasic/Constant  const=L2N  gui_display_data_type=Fixed-point  arith_type=Unsigned  n_bits=ceil(log2(L2M+L2N))  bin_pt=0  preci_type=Single  exp_width=8  frac_width=24  explicit_period=on  period=1  XmcBlockStatus=1  maskContainerNames=tabcontainer1  block_type=constant  block_config=sysgen:Constant_config
  Constant4 : hdlBasic/Constant  const=L2M  gui_display_data_type=Fixed-point  arith_type=Unsigned  n_bits=ceil(log2(L2M+L2N))  bin_pt=0  preci_type=Single  exp_width=8  frac_width=24  explicit_period=on  period=1  XmcBlockStatus=1  maskContainerNames=tabcontainer1  block_type=constant  block_config=sysgen:Constant_config
  Constant5 : hdlBasic/Constant  const=2^ceil(log2(L2M+L2N))-L2M  gui_display_data_type=Fixed-point  arith_type=Unsigned  n_bits=ceil(log2(L2M+L2N))  bin_pt=0  preci_type=Single  exp_width=8  frac_width=24  explicit_period=on  period=1  XmcBlockStatus=1  maskContainerNames=tabcontainer1  block_type=constant  block_config=sysgen:Constant_config
  Mux : hdlBasic/Mux  inputs=2  en=off  latency=0  precision=Full  arith_type=Unsigned  n_bits=16  bin_pt=14  quantization=Truncate  overflow=Wrap  XmcBlockStatus=1  maskContainerNames=tabcontainer1  block_type=mux  block_config=sysgen:Mux_config
  Register : hdlBasic/Register  init=L2N  rst=off  en=on  XmcBlockStatus=1  maskContainerNames=tabcontainer1  block_type=register  block_config=sysgen:Register_config
  Relational1 : hdlBasic/Relational  mode=a>=b  op_type=Bool  en=off  latency=0  XmcBlockStatus=1  maskContainerNames=tabcontainer1  block_type=relational  block_config=sysgen:Relational_config
  O : Outport
  wires:
  EN/1 -> Register/2
  Constant4/1 -> Relational1/2
  AddSub/1 -> Register/1
  Constant5/1 -> Mux/3
  Constant1/1 -> Mux/2
  Mux/1 -> AddSub/2
  Relational1/1 -> Mux/1
  Register/1 -> Relational1/1, AddSub/1, O/1

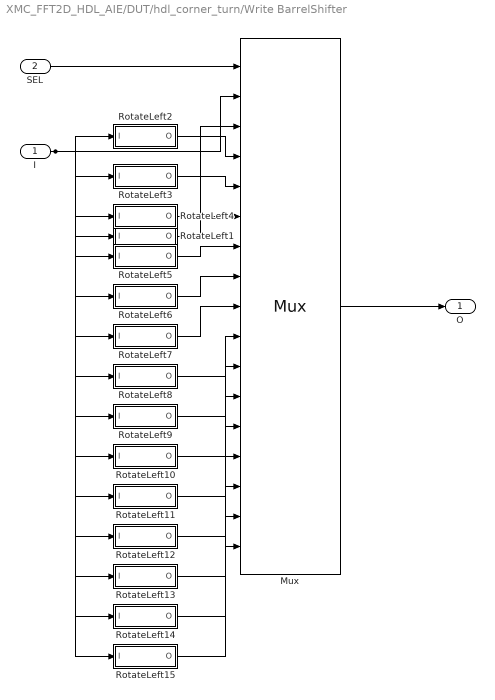
== system XMC_FFT2D_HDL_AIE/DUT/hdl_corner_turn/Write BarrelShifter ==
  I : Inport
  SEL : Inport  Port=2
  Mux : hdlBasic/Mux  inputs=16  en=off  latency=1  precision=Full  arith_type=Unsigned  n_bits=16  bin_pt=14  quantization=Truncate  overflow=Wrap  XmcBlockStatus=1  maskContainerNames=tabcontainer1  block_type=mux  block_config=sysgen:Mux_config
  RotateLeft1 : Subsystem  mask{NB=1, W=barrel_length}
      mask prompts: NB "Number of bits (cannot be 0):"; W "Width"
  RotateLeft10 : Subsystem  mask{NB=10, W=barrel_length}
      mask prompts: NB "Number of bits (cannot be 0):"; W "Width"
  RotateLeft11 : Subsystem  mask{NB=11, W=barrel_length}
      mask prompts: NB "Number of bits (cannot be 0):"; W "Width"
  RotateLeft12 : Subsystem  mask{NB=12, W=barrel_length}
      mask prompts: NB "Number of bits (cannot be 0):"; W "Width"
  RotateLeft13 : Subsystem  mask{NB=13, W=barrel_length}
      mask prompts: NB "Number of bits (cannot be 0):"; W "Width"
  RotateLeft14 : Subsystem  mask{NB=14, W=barrel_length}
      mask prompts: NB "Number of bits (cannot be 0):"; W "Width"
  RotateLeft15 : Subsystem  mask{NB=15, W=barrel_length}
      mask prompts: NB "Number of bits (cannot be 0):"; W "Width"
  RotateLeft2 : Subsystem  mask{NB=2, W=barrel_length}
      mask prompts: NB "Number of bits (cannot be 0):"; W "Width"
  RotateLeft3 : Subsystem  mask{NB=3, W=barrel_length}
      mask prompts: NB "Number of bits (cannot be 0):"; W "Width"
  RotateLeft4 : Subsystem  mask{NB=4, W=barrel_length}
      mask prompts: NB "Number of bits (cannot be 0):"; W "Width"
  RotateLeft5 : Subsystem  mask{NB=5, W=barrel_length}
      mask prompts: NB "Number of bits (cannot be 0):"; W "Width"
  RotateLeft6 : Subsystem  mask{NB=6, W=barrel_length}
      mask prompts: NB "Number of bits (cannot be 0):"; W "Width"
  RotateLeft7 : Subsystem  mask{NB=7, W=barrel_length}
      mask prompts: NB "Number of bits (cannot be 0):"; W "Width"
  RotateLeft8 : Subsystem  mask{NB=8, W=barrel_length}
      mask prompts: NB "Number of bits (cannot be 0):"; W "Width"
  RotateLeft9 : Subsystem  mask{NB=9, W=barrel_length}
      mask prompts: NB "Number of bits (cannot be 0):"; W "Width"
  O : Outport
  wires:
  RotateLeft1/1(O) -> Mux/3
  RotateLeft2/1(O) -> Mux/4
  RotateLeft3/1(O) -> Mux/5
  RotateLeft4/1(O) -> Mux/6
  RotateLeft5/1(O) -> Mux/7
  RotateLeft6/1(O) -> Mux/8
  RotateLeft7/1(O) -> Mux/9
  RotateLeft8/1(O) -> Mux/10
  RotateLeft9/1(O) -> Mux/11
  RotateLeft10/1(O) -> Mux/12
  RotateLeft11/1(O) -> Mux/13
  RotateLeft12/1(O) -> Mux/14
  RotateLeft13/1(O) -> Mux/15
  RotateLeft14/1(O) -> Mux/16
  RotateLeft15/1(O) -> Mux/17
  Mux/1 -> O/1
  I/1 -> RotateLeft1/1(I), RotateLeft2/1(I), RotateLeft3/1(I), RotateLeft4/1(I), RotateLeft5/1(I), RotateLeft6/1(I), RotateLeft7/1(I), RotateLeft8/1(I), RotateLeft9/1(I), RotateLeft10/1(I), RotateLeft11/1(I), RotateLeft12/1(I), RotateLeft13/1(I), RotateLeft14/1(I), RotateLeft15/1(I), Mux/2
  SEL/1 -> Mux/1

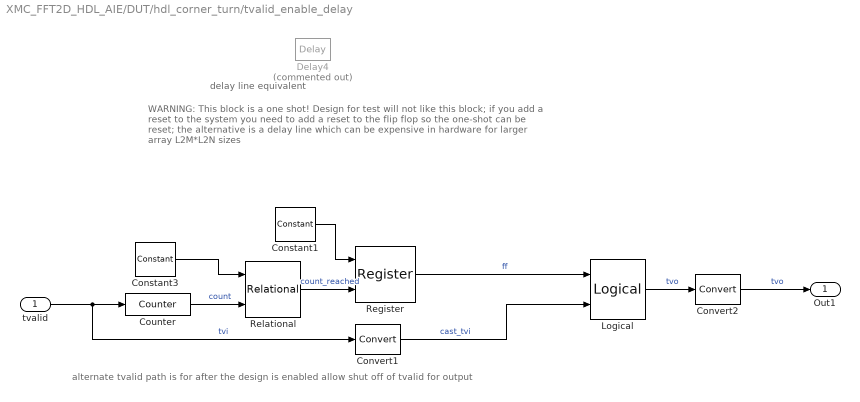
== system XMC_FFT2D_HDL_AIE/DUT/hdl_corner_turn/tvalid_enable_delay ==
  note: alternate tvalid path is for after the design is enabled allow shut off of tvalid for output
  note: delay line equivalent
  note: WARNING: This block is a one shot! Design for test will not like this block; if you add a reset to the system you need to add a reset to the flip flop so the one-shot can be reset; the alternative is a delay line which can be expensive in hardware for larger array L2M*L2N sizes
  tvalid : Inport
  Constant1 : hdlBasic/Constant  const=1  gui_display_data_type=Fixed-point  arith_type=Unsigned  n_bits=1  bin_pt=0  preci_type=Single  exp_width=8  frac_width=24  explicit_period=off  period=1  XmcBlockStatus=1  maskContainerNames=tabcontainer1  block_type=constant  block_config=sysgen:Constant_config
  Constant3 : hdlBasic/Constant  const=2^(L2M+L2N)-(2^L2M+2^L2N)+1  gui_display_data_type=Fixed-point  arith_type=Unsigned  n_bits=L2M+L2N  bin_pt=0  preci_type=Single  exp_width=8  frac_width=24  explicit_period=off  period=1  XmcBlockStatus=1  maskContainerNames=tabcontainer1  block_type=constant  block_config=sysgen:Constant_config
  Convert1 : hdlBasic/Convert  gui_display_data_type=Fixed-point  arith_type=Unsigned  n_bits=1  bin_pt=0  float_type=Single  exp_bits=8  fraction_bits=24  quantization=Truncate  overflow=Wrap  en=off  latency=0  pipeline=off  XmcBlockStatus=1  maskContainerNames=group2  block_type=convert  block_config=sysgen:Convert_config  block_width=595  block_height=885
  Convert2 : hdlBasic/Convert  gui_display_data_type=Boolean  arith_type=Boolean  n_bits=1  bin_pt=0  float_type=Single  exp_bits=8  fraction_bits=24  quantization=Truncate  overflow=Wrap  en=off  latency=0  pipeline=off  XmcBlockStatus=1  maskContainerNames=group2  block_type=convert  block_config=sysgen:Convert_config  block_width=595  block_height=885
  Counter : hdlBasic/Counter  cnt_type=Count limited  cnt_to=2^(L2M+L2N)-(2^L2M+2^L2N)+2  operation=Up  start_count=0  cnt_by_val=1  arith_type=Unsigned  n_bits=L2M+L2N  bin_pt=0  load_pin=off  rst=off  en=on  explicit_period=Explicit  period=1  use_behavioral_HDL=off  implementation=Fabric  XmcBlockStatus=1  maskContainerNames=group1  block_type=counter  block_config=sysgen:Counter_config  block_width=531  block_height=1023
  Delay4 : hdlBasic/Delay  Commented=on  rst=off  en=off  latency=2^(L2M+L2N)-(2^L2M+2^L2N)+2  reg_retiming=off  XmcBlockStatus=1  maskContainerNames=group1  block_type=delay  block_config=sysgen:Delay_config
  Logical : hdlBasic/Logical  logical_function=AND  inputs=2  en=off  latency=1  precision=Full  arith_type=Unsigned  n_bits=16  bin_pt=0  align_bp=on  overflow=[]  quantization=[]  XmcBlockStatus=1  maskContainerNames=tabcontainer1  block_type=logical  block_config=sysgen:Logical_config
  Register : hdlBasic/Register  init=0  rst=off  en=on  XmcBlockStatus=1  maskContainerNames=tabcontainer1  block_type=register  block_config=sysgen:Register_config
  Relational : hdlBasic/Relational  mode=a=b  op_type=Bool  en=off  latency=0  XmcBlockStatus=1  maskContainerNames=tabcontainer1  block_type=relational  block_config=sysgen:Relational_config
  Out1 : Outport
  wires:
  Register/1 -> Logical/1  "ff"
  tvalid/1 -> Counter/1, Convert1/1  "tvi"
  Counter/1 -> Relational/2  "count"
  Relational/1 -> Register/2  "count_reached"
  Convert2/1 -> Out1/1  "tvo"
  Constant3/1 -> Relational/1
  Convert1/1 -> Logical/2  "cast_tvi"
  Constant1/1 -> Register/1
  Logical/1 -> Convert2/1  "tvo"

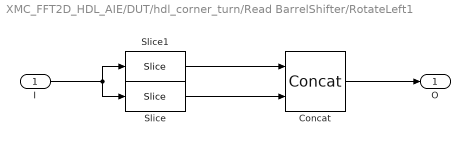
== system XMC_FFT2D_HDL_AIE/DUT/hdl_corner_turn/Read BarrelShifter/RotateLeft1 ==
  I : Inport
  Concat : hdlBasic/Concat  num_inputs=2  XmcBlockStatus=1  maskContainerNames=group1  block_type=concat  block_config=sysgen:Concat_config
  Slice : hdlBasic/Slice  nbits=NB  boolean_output=off  mode=Upper Bit Location + Width  bit1=0  base1=MSB of Input  bit0=0  base0=LSB of Input  XmcBlockStatus=1  maskContainerNames=group1  block_type=slice  block_config=sysgen:Slice_config
  Slice1 : hdlBasic/Slice  nbits=W-NB  boolean_output=off  mode=Lower Bit Location + Width  bit1=0  base1=MSB of Input  bit0=0  base0=LSB of Input  XmcBlockStatus=1  maskContainerNames=group1  block_type=slice  block_config=sysgen:Slice_config
  O : Outport
  wires:
  Slice1/1 -> Concat/1
  Slice/1 -> Concat/2
  Concat/1 -> O/1
  I/1 -> Slice/1, Slice1/1

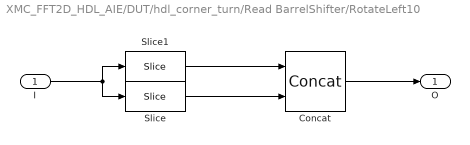
== system XMC_FFT2D_HDL_AIE/DUT/hdl_corner_turn/Read BarrelShifter/RotateLeft10 ==
  I : Inport
  Concat : hdlBasic/Concat  num_inputs=2  XmcBlockStatus=1  maskContainerNames=group1  block_type=concat  block_config=sysgen:Concat_config
  Slice : hdlBasic/Slice  nbits=NB  boolean_output=off  mode=Upper Bit Location + Width  bit1=0  base1=MSB of Input  bit0=0  base0=LSB of Input  XmcBlockStatus=1  maskContainerNames=group1  block_type=slice  block_config=sysgen:Slice_config
  Slice1 : hdlBasic/Slice  nbits=W-NB  boolean_output=off  mode=Lower Bit Location + Width  bit1=0  base1=MSB of Input  bit0=0  base0=LSB of Input  XmcBlockStatus=1  maskContainerNames=group1  block_type=slice  block_config=sysgen:Slice_config
  O : Outport
  wires:
  I/1 -> Slice1/1, Slice/1
  Concat/1 -> O/1
  Slice/1 -> Concat/2
  Slice1/1 -> Concat/1

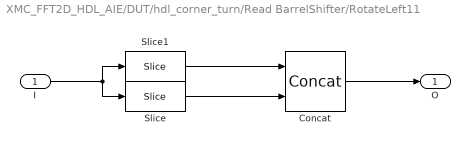
== system XMC_FFT2D_HDL_AIE/DUT/hdl_corner_turn/Read BarrelShifter/RotateLeft11 ==
  I : Inport
  Concat : hdlBasic/Concat  num_inputs=2  XmcBlockStatus=1  maskContainerNames=group1  block_type=concat  block_config=sysgen:Concat_config
  Slice : hdlBasic/Slice  nbits=NB  boolean_output=off  mode=Upper Bit Location + Width  bit1=0  base1=MSB of Input  bit0=0  base0=LSB of Input  XmcBlockStatus=1  maskContainerNames=group1  block_type=slice  block_config=sysgen:Slice_config
  Slice1 : hdlBasic/Slice  nbits=W-NB  boolean_output=off  mode=Lower Bit Location + Width  bit1=0  base1=MSB of Input  bit0=0  base0=LSB of Input  XmcBlockStatus=1  maskContainerNames=group1  block_type=slice  block_config=sysgen:Slice_config
  O : Outport
  wires:
  I/1 -> Slice1/1, Slice/1
  Concat/1 -> O/1
  Slice/1 -> Concat/2
  Slice1/1 -> Concat/1

== system XMC_FFT2D_HDL_AIE/DUT/hdl_corner_turn/Read BarrelShifter/RotateLeft12 ==
  I : Inport
  Concat : hdlBasic/Concat  num_inputs=2  XmcBlockStatus=1  maskContainerNames=group1  block_type=concat  block_config=sysgen:Concat_config
  Slice : hdlBasic/Slice  nbits=NB  boolean_output=off  mode=Upper Bit Location + Width  bit1=0  base1=MSB of Input  bit0=0  base0=LSB of Input  XmcBlockStatus=1  maskContainerNames=group1  block_type=slice  block_config=sysgen:Slice_config
  Slice1 : hdlBasic/Slice  nbits=W-NB  boolean_output=off  mode=Lower Bit Location + Width  bit1=0  base1=MSB of Input  bit0=0  base0=LSB of Input  XmcBlockStatus=1  maskContainerNames=group1  block_type=slice  block_config=sysgen:Slice_config
  O : Outport
  wires:
  I/1 -> Slice1/1, Slice/1
  Concat/1 -> O/1
  Slice/1 -> Concat/2
  Slice1/1 -> Concat/1

== system XMC_FFT2D_HDL_AIE/DUT/hdl_corner_turn/Read BarrelShifter/RotateLeft13 ==
  I : Inport
  Concat : hdlBasic/Concat  num_inputs=2  XmcBlockStatus=1  maskContainerNames=group1  block_type=concat  block_config=sysgen:Concat_config
  Slice : hdlBasic/Slice  nbits=NB  boolean_output=off  mode=Upper Bit Location + Width  bit1=0  base1=MSB of Input  bit0=0  base0=LSB of Input  XmcBlockStatus=1  maskContainerNames=group1  block_type=slice  block_config=sysgen:Slice_config
  Slice1 : hdlBasic/Slice  nbits=W-NB  boolean_output=off  mode=Lower Bit Location + Width  bit1=0  base1=MSB of Input  bit0=0  base0=LSB of Input  XmcBlockStatus=1  maskContainerNames=group1  block_type=slice  block_config=sysgen:Slice_config
  O : Outport
  wires:
  I/1 -> Slice1/1, Slice/1
  Concat/1 -> O/1
  Slice/1 -> Concat/2
  Slice1/1 -> Concat/1
